simulink model "Project_sinePWM_example"  (R2020a)
settings: Solver=ode4  StartTime=0  StopTime=1  FixedStep=5e-6  MaxStep=1e-6  RelTol=1e-6  AbsTol=1e-6  EnableMultiTasking=on
PreLoadFcn:
  | assignin('base','Ts',[5e-6])
libraries: powerlib x14, powerlib_meascontrol x3
Description:
  | This example illustrates use of the BLDC in a closed-loop
  | speed and voltage control on a 1 kW, 3000 rpm industrial motor
  | 
  | 
  | Copyright 2008-2017 The MathWorks, Inc.
settings Model: ExtModeAutoUpdateStatusClock=off  Creator=MathWorks  LastModifiedBy=gapaul
settings SolverCC: AutoScaleAbsTol=off
settings DataIOCC: LimitDataPoints=on  SaveFormat=Array  SignalLoggingSaveFormat=ModelDataLogs  ReturnWorkspaceOutputs=off  SignalLoggingName=sigsOut
settings OptimizationCC: ExpressionDepthLimit=2147483647  InitFltsAndDblsToZero=on  LifeSpan=inf
settings DebuggingCC: UnderspecifiedInitializationDetection=Classic  MergeDetectMultiDrivingBlocksExec=none  SignalResolutionControl=TryResolveAllWithWarning  MultiTaskDSMMsg=warning  MultiTaskCondExecSysMsg=none  FcnCallInpInsideContextMsg=warning  StateNameClashWarn=warning  SFUnexpectedBacktrackingDiag=warning  SFNoUnconditionalDefaultTransitionDiag=warning  SFExecutionAtInitializationDiag=none  ArithmeticOperatorsInVariantConditions=warning
settings HardwareCC: ProdBitPerPointer=32  ProdBitPerSizeT=32  ProdBitPerPtrDiffT=32  ProdLargestAtomicFloat=None  ProdIntDivRoundTo=Undefined  ProdEndianess=Unspecified  ProdWordSize=32  ProdHWDeviceType=32-bit Generic  TargetUnknown=on
settings ModelReferenceCC: PropagateSignalLabelsOutOfModel=off
settings SFSimCC: SimUseLocalCustomCode=off  CustomCodeUndefinedFunction=UseInterfaceOnly
settings RTWCC: RTWUseLocalCustomCode=off
settings CodeAppCC: StateflowObjectComments=on
settings GRTTargetCC: TargetLangStandard=C89/C90 (ANSI)  CombineOutputUpdateFcns=off  GRTInterface=on
settings ConfigComp: CovMetricSettings=dw  CovHtmlReporting=on  CovSaveCumulativeToWorkspaceVar=on  CovSaveSingleToWorkspaceVar=on  CovExternalEMLEnable=off  CovSFcnEnable=off
settings SimscapeCC: SimscapeNormalizeSystem=off

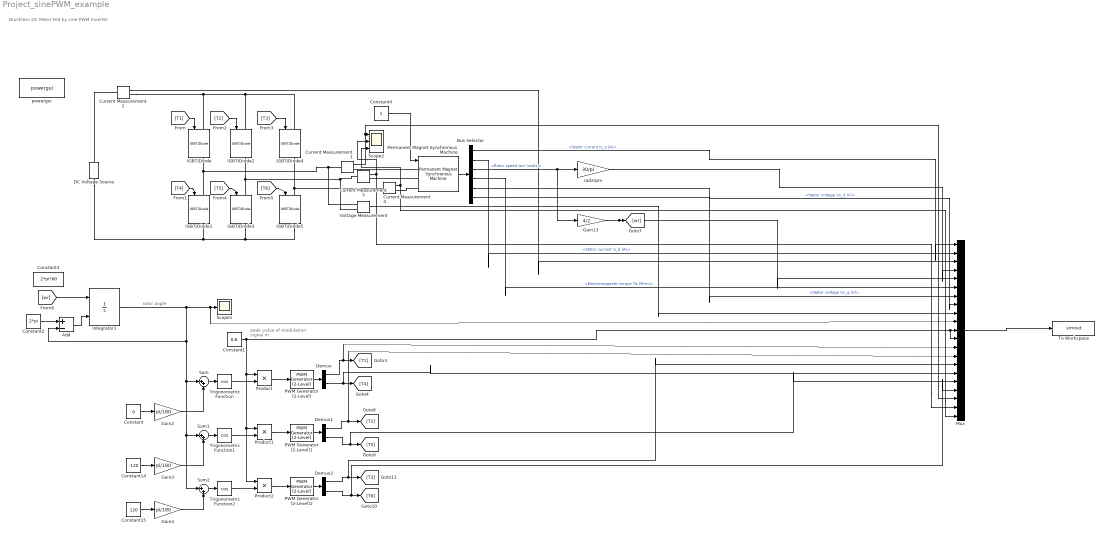
== system Project_sinePWM_example ==
  note: peak value of modulation signal m
  note: Brushless DC Motor Fed by sine PWM Inverter
  note: rotor angle
  Add : Sum  Inputs=+-
  Bus Selector : BusSelector  OutputSignals=Stator current is_q (A),Stator current is_d (A),Rotor speed wm (rad/s),Electromagnetic torque Te (N*m),Stator voltage Vs_q (V),Stator voltage Vs_d (V)
  Constant : Constant  Value=0
  Constant1 : Constant  Value=0.6
  Constant14 : Constant  Value=-120
  Constant15 : Constant  Value=120
  Constant2 : Constant  Value=2*pi
  Constant3 : Constant  Value=2*pi*60
  Constant4 : Constant
  Current Measurement{1..4} (4 alike) : powerlib/Measurements/Current Measurement  PhasorSimulation=off  OutputType=Complex  PSBequivalent=0
  DC Voltage Source : powerlib/Electrical Sources/DC Voltage Source  Amplitude=72  Measurements=None
  Demux : Demux  Outputs=2
  Demux1 : Demux  Outputs=2
  Demux2 : Demux  Outputs=2
  Gain13 : Gain  Gain=4/2
  Gain2 : Gain  Gain=pi/180
  Gain3 : Gain  Gain=pi/180
  Gain4 : Gain  Gain=pi/180
  IGBT/Diode{,1..5} (6 alike) : powerlib/Power Electronics/IGBT//Diode  Ron=1e-5  Rs=1e5  Cs=inf  Measurements=on
  Integrator1 : Integrator  ExternalReset=falling
  Mux : Mux  Inputs=21
  PWM Generator (2-Level) : powerlib_meascontrol/Pulse & Signal Generators/PWM Generator (2-Level)  ModulatorType=Single-phase half-bridge (2 pulses)  ModulatorMode=Unsynchronized  Fc=1620  Pc=90  nF=30  MinMax="[ -1  1 ]"  SamplingTechnique=Natural  ModulatingSignals=off  m=0.8  Freq=60  Phase=0  Ts=5e-6  ShowCarrierOutport=off
  PWM Generator (2-Level)1 : powerlib_meascontrol/Pulse & Signal Generators/PWM Generator (2-Level)  ModulatorType=Single-phase half-bridge (2 pulses)  ModulatorMode=Unsynchronized  Fc=1620  Pc=90  nF=30  MinMax="[ -1  1 ]"  SamplingTechnique=Natural  ModulatingSignals=off  m=0.8  Freq=60  Phase=0  Ts=5e-6  ShowCarrierOutport=off
  PWM Generator (2-Level)2 : powerlib_meascontrol/Pulse & Signal Generators/PWM Generator (2-Level)  ModulatorType=Single-phase half-bridge (2 pulses)  ModulatorMode=Unsynchronized  Fc=1620  Pc=90  nF=30  MinMax="[ -1  1 ]"  SamplingTechnique=Natural  ModulatingSignals=off  m=0.8  Freq=60  Phase=0  Ts=5e-6  ShowCarrierOutport=off
  Permanent Magnet Synchronous Machine : powerlib/Machines/Permanent Magnet Synchronous Machine  NbPhases=3  FluxDistribution=Sinusoidal  RotorType=Round  MechanicalLoad=Torque Tm  PresetModel=No  ShowDetailedParameters=on  MeasurementBus=off  Resistance=3.4  Inductance=8.5e-3  dqInductances=[8.5e-3, 8.5e-3]  La=(1.1 + 3/2*11)*1e-3  MachineConstant=Flux linkage established by magnets (V.s)  Flux=0.2  VoltageCst=72.552  TorqueCst=0.6  Flat=120  Mechanical=[5e-4, 0 2]  PolePairs=4  InitialConditions=[0,0, 0,0]  InitialConditions5ph=[0 0 0 0 0 0]  RefAngle=90 degrees behind phase A axis (modified Park)  IterativeDiscreteModel=Trapezoidal non iterative  TsBlock=-1  TsPowergui=0
  Product : Product
  Product1 : Product
  Product2 : Product
  Scope1 : Scope
  Scope2 : Scope  NumInputPorts=3
  Sum : Sum  Inputs=|++
  Sum1 : Sum  Inputs=|++
  Sum2 : Sum  Inputs=|++
  To Workspace : ToWorkspace  VariableName=simout  SaveFormat=Timeseries  SampleTime=-1
  Trigonometric Function : Trigonometry  Operator=cos
  Trigonometric Function1 : Trigonometry  Operator=cos
  Trigonometric Function2 : Trigonometry  Operator=cos
  Voltage Measurement : powerlib/Measurements/Voltage Measurement  PhasorSimulation=off  OutputType=Complex  PSBequivalent=0
  powergui : powerlib/powergui  Priority=2  SimulationMode=Discrete  SampleTime=5e-6  frequency=60  Iterations=50  frequencyindice=0  Pbase=100e6  ErrMax=1e-4  UnitsV=kV  UnitsW=MW  buscounter=0  FunctionMessages=off  echomessages=off  EnableUseOfTLC=off  CurrentSourceSwitches=off  DisableSnubberDevices=off  DisableRonSwitches=off  DisableVfSwitches=off  DisplayEquations=off  AutomaticDiscreteSolvers=off  SolverType=Tustin/Backward Euler (TBE)  Interpol=off  ExternalGateDelay=off  methode=off  Ts=0  x0status=blocks  SPID=off  SwTol=0  HookPort=off  NonlinearTolerance=1e-4  nMaxIteration=100  ContinueOnMaxIteration=off  RestoreLinks=warning  ResistiveCurrentMeasurement=off  Frange=[0:2:500]  Ylog=off  Xlog=on  ShowGrid=off  save=off  variable=ZData  structure=0  ZoomFFT=on  StartTime=0.0  cycles=1  DisplayStyle=1  fundamental=60  FreqAxis=off  MaxFrequency=1000  frequencyindicesteady=1  RmsSteady=1  display=off
  rad2rpm : Gain  Gain=30/pi
  wires:
  Constant4/1 -> Permanent Magnet Synchronous Machine/1
  Voltage Measurement/1 -> Mux/9
  Permanent Magnet Synchronous Machine/1 -> Bus Selector/1
  Bus Selector/3 -> Gain13/1, rad2rpm/1  "<Rotor speed wm (rad/s)>"
  Bus Selector/2 -> Mux/2  "<Stator current is_d (A)>"
  [T4] -> IGBT/Diode1/1
  [T5] -> IGBT/Diode3/1
  [T6] -> IGBT/Diode5/1
  [T1] -> IGBT/Diode/1
  [T2] -> IGBT/Diode2/1
  [T3] -> IGBT/Diode4/1
  Constant2/1 -> Add/1
  Add/1 -> Integrator1/2
  [wr] -> Integrator1/1
  Bus Selector/6 -> Mux/8  "<Stator voltage Vs_d (V)>"
  Constant/1 -> Gain2/1
  PWM Generator (2-Level)1/1 -> Demux1/1
  PWM Generator (2-Level)2/1 -> Demux2/1
  Sum1/1 -> Trigonometric Function1/1
  Gain3/1 -> Sum1/2
  Sum/1 -> Trigonometric Function/1
  Gain4/1 -> Sum2/2
  Constant14/1 -> Gain3/1
  Constant15/1 -> Gain4/1
  Gain2/1 -> Sum/2
  Sum2/1 -> Trigonometric Function2/1
  Product2/1 -> PWM Generator (2-Level)2/1
  Product/1 -> PWM Generator (2-Level)/1
  Product1/1 -> PWM Generator (2-Level)1/1
  Trigonometric Function2/1 -> Product2/2
  Trigonometric Function1/1 -> Product1/2
  Trigonometric Function/1 -> Product/2
  Demux/1 -> Mux/13, [T1]
  Demux/2 -> Mux/16, [T4]
  Demux2/2 -> Mux/18, [T6]
  Current Measurement4/1 -> Mux/21, Scope2/3
  Current Measurement2/1 -> Mux/3
  Bus Selector/5 -> Mux/7  "<Stator voltage Vs_q (V)>"
  Current Measurement1/1 -> Mux/19, Scope2/1
  Integrator1/1 -> Mux/10, Scope1/1, Add/2, Sum/1, Sum2/1, Sum1/1
  Demux1/2 -> Mux/17, [T5]
  rad2rpm/1 -> Mux/4
  Constant1/1 -> Mux/12, Mux/11, Product2/1, Product1/1, Product/1
  Gain13/1 -> Mux/5, [wr]
  Demux2/1 -> Mux/15, [T3]
  Current Measurement3/1 -> Mux/20, Scope2/2
  PWM Generator (2-Level)/1 -> Demux/1
  Bus Selector/1 -> Mux/1  "<Stator current is_q (A)>"
  Demux1/1 -> Mux/14, [T2]
  Bus Selector/4 -> Mux/6  "<Electromagnetic torque Te (N*m)>"
  Mux/1 -> To Workspace/1
  connections:
  IGBT/Diode/RConn1 -- Current Measurement1/LConn1 -- Voltage Measurement/LConn1 -- IGBT/Diode1/LConn1
  IGBT/Diode2/RConn1 -- Current Measurement3/LConn1 -- Voltage Measurement/LConn2 -- IGBT/Diode3/LConn1
  IGBT/Diode4/RConn1 -- Current Measurement4/LConn1 -- IGBT/Diode5/LConn1
  IGBT/Diode1/RConn1 -- DC Voltage Source/LConn1 -- IGBT/Diode5/RConn1 -- IGBT/Diode3/RConn1
  IGBT/Diode2/LConn1 -- IGBT/Diode4/LConn1 -- IGBT/Diode/LConn1 -- Current Measurement2/RConn1
  Current Measurement2/LConn1 -- DC Voltage Source/RConn1
  Current Measurement1/RConn1 -- Permanent Magnet Synchronous Machine/LConn1
  Current Measurement3/RConn1 -- Permanent Magnet Synchronous Machine/LConn2
  Current Measurement4/RConn1 -- Permanent Magnet Synchronous Machine/LConn3
